simulink model "D4_O_full_wave_rectifier_circuit"  (R2021b)
settings: Solver=VariableStepAuto  StartTime=0.0  StopTime=0.1  MaxStep=0.0001  RelTol=1e-3
libraries: spsDiodeLib x4, spsSeriesRLCBranchLib x3, spsMultimeterLib x3, spsACVoltageSourceLib x1, spsBreakerLib x1, spspowerguiLib x1
settings Model: Creator=12481  LastModifiedBy=12481

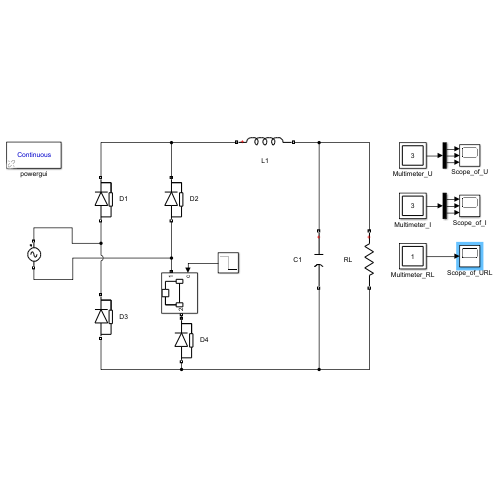
[thumbnail: Simulink's stored preview of the top-level diagram]
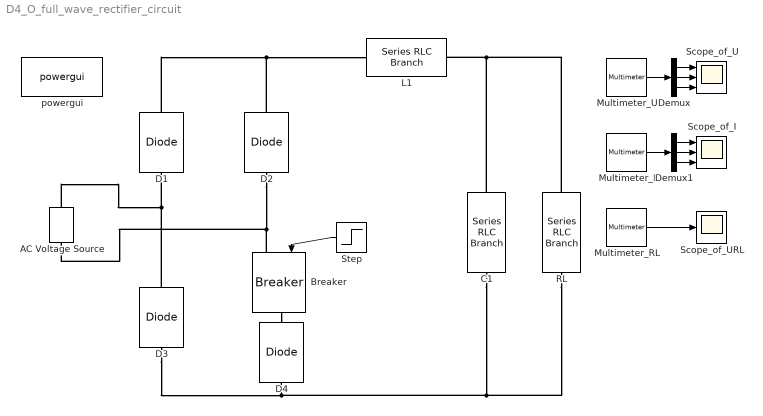
== system D4_O_full_wave_rectifier_circuit ==
  AC Voltage Source : spsACVoltageSourceLib/AC Voltage Source  Amplitude=220*sqrt(2)  Phase=0  Frequency=50  SampleTime=0  Measurements=None  BusType=swing  Pref=10e3  Qref=0  Qmin=-inf  Qmax=+inf
  Breaker : spsBreakerLib/Breaker  InitialState=1  SwitchingTimes="[1/60  5/60]"  External=on  BreakerResistance=0.0001  SnubberResistance=1e6  SnubberCapacitance=inf  Measurements=None  MoreParameters=on  NoBreakLoop=off
      settings: SourceProductBaseCode=PS
  C1 : spsSeriesRLCBranchLib/Series RLC Branch  LConnTagsString=__new0  RConnTagsString=__new0  BranchType=C  Resistance=1  Inductance=1e-3  SetiL0=off  InitialCurrent=0  Capacitance=4700e-6  Setx0=off  InitialVoltage=0  Measurements=Branch voltage and current
  D{1..4} (4 alike) : spsDiodeLib/Diode  Ron=0.001  Lon=0  Vf=0.8  IC=0  UseSnubber=0  Rs=500  Cs=250e-9  Measurements=off
  Demux : Demux  Outputs=3
  Demux1 : Demux  Outputs=3
  L1 : spsSeriesRLCBranchLib/Series RLC Branch  LConnTagsString=__new0  RConnTagsString=__new0  BranchType=L  Resistance=1  Inductance=10e-3  SetiL0=off  InitialCurrent=0  Capacitance=1e-6  Setx0=off  InitialVoltage=0  Measurements=Branch voltage and current
  Multimeter_I : spsMultimeterLib/Multimeter  PhasorSimulation=off  OutputType=Complex  sel=[5 4 6]  L=6  Gain=[1 1 1]  yselected={'Ib: L1','Ib: C1','Ib: RL'};  PSBOutputType=1  PSBequivalent=0  AxesSetting=[0,0.1,-100,100]  Display=0  SavedBlockNames=-11
  Multimeter_RL : spsMultimeterLib/Multimeter  PhasorSimulation=off  OutputType=Complex  sel=3  L=6  Gain=1  yselected={'Ub: RL'};  PSBOutputType=1  PSBequivalent=0  AxesSetting=[0,0.1,-100,100]  Display=0  SavedBlockNames=-11
  Multimeter_U : spsMultimeterLib/Multimeter  PhasorSimulation=off  OutputType=Complex  sel=[2 1 3]  L=6  Gain=[1 1 1]  yselected={'Ub: L1','Ub: C1','Ub: RL'};  PSBOutputType=1  PSBequivalent=0  AxesSetting=[0,0.1,-100,100]  Display=0  SavedBlockNames=-11
  RL : spsSeriesRLCBranchLib/Series RLC Branch  LConnTagsString=__new0  RConnTagsString=__new0  BranchType=R  Resistance=1  Inductance=1e-3  SetiL0=off  InitialCurrent=0  Capacitance=1e-6  Setx0=off  InitialVoltage=0  Measurements=Branch voltage and current
  Scope_of_I : Scope  NumInputPorts=3
  Scope_of_U : Scope  NumInputPorts=3
  Scope_of_URL : Scope
  Step : Step  Time=0.04  Before=1  After=0  SampleTime=0
  powergui : spspowerguiLib/powergui  Priority=1  SimulationMode=Continuous  SampleTime=50e-6  frequency=60  Iterations=50  frequencyindice=50  Pbase=100e6  ErrMax=1e-4  UnitsV=kV  UnitsW=MW  buscounter=0  FunctionMessages=off  echomessages=off  EnableUseOfTLC=off  CurrentSourceSwitches=off  DisableSnubberDevices=off  DisableRonSwitches=off  DisableVfSwitches=off  DisplayEquations=off  AutomaticDiscreteSolvers=off  SolverType=Tustin/Backward Euler (TBE)  Interpol=off  ExternalGateDelay=off  methode=off  Ts=100  x0status=blocks  SPID=on  SwTol=0  HookPort=off  NonlinearTolerance=1e-4  nMaxIteration=100  ContinueOnMaxIteration=off  RestoreLinks=warning  ResistiveCurrentMeasurement=off  Frange=[0:2:500]  Ylog=off  Xlog=on  ShowGrid=off  save=off  variable=ZData  structure=0  ZoomFFT=off  StartTime=0.0  cycles=1  DisplayStyle=1  fundamental=60  FreqAxis=off  MaxFrequency=1000  frequencyindicesteady=1  RmsSteady=1  display=off
  wires:
  Multimeter_U/1 -> Demux/1
  Multimeter_I/1 -> Demux1/1
  Demux/1 -> Scope_of_U/1
  Demux/2 -> Scope_of_U/2
  Demux/3 -> Scope_of_U/3
  Demux1/1 -> Scope_of_I/1
  Demux1/2 -> Scope_of_I/2
  Demux1/3 -> Scope_of_I/3
  Multimeter_RL/1 -> Scope_of_URL/1
  Step/1 -> Breaker/1
  connections:
  AC Voltage Source/RConn1 -- D1/LConn1 -- D3/RConn1
  D1/RConn1 -- L1/LConn1 -- D2/RConn1
  C1/RConn1 -- RL/RConn1 -- D3/LConn1 -- D4/LConn1
  RL/LConn1 -- C1/LConn1 -- L1/RConn1
  D2/LConn1 -- Breaker/LConn1 -- AC Voltage Source/LConn1
  Breaker/RConn1 -- D4/RConn1
